simulink model "power_dstatcom_pwm"  (R2013a)
settings: Solver=FixedStepDiscrete  SolverMode=SingleTasking  StartTime=0.0  StopTime=0.5  FixedStep=Ts  RelTol=1e-3
InitFcn:
  |  Ts=5e-6;
undefined symbols (not defined in the file): D11, Delta, DiscIntNeverNeededParam
libraries: powerlib x39, powerlib_extras x25
(part 1 of 2)
Description:
  | Copyright 2008-2013 The MathWorks, Inc.
settings Model: ExtModeTrigMode=oneshot  ExtModeArmWhenConnect=off  ExtModeAutoUpdateStatusClock=off  Creator=MathWorks  LastModifiedBy=nau03113
settings DataIOCC: LimitDataPoints=off  SaveFinalState=on  SaveFormat=Structure  SignalLoggingSaveFormat=ModelDataLogs  SaveOutput=off  SaveTime=off  SignalLoggingName=sigsOut
settings OptimizationCC: BlockReduction=off  BooleanDataType=off  ExpressionDepthLimit=2147483647  InitFltsAndDblsToZero=on
settings DebuggingCC: SaveWithParameterizedLinksMsg=none  SignalResolutionControl=TryResolveAllWithWarning  SolverPrmCheckMsg=none  MultiTaskDSMMsg=warning  MultiTaskCondExecSysMsg=none  FcnCallInpInsideContextMsg=UseLocalSettings
settings HardwareCC: TargetUnknown=on
settings RTWCC: IncludeERTFirstTime=on
settings GRTTargetCC: TargetFcnLib=ansi_tfl_tmw.mat  CombineOutputUpdateFcns=off  GRTInterface=on

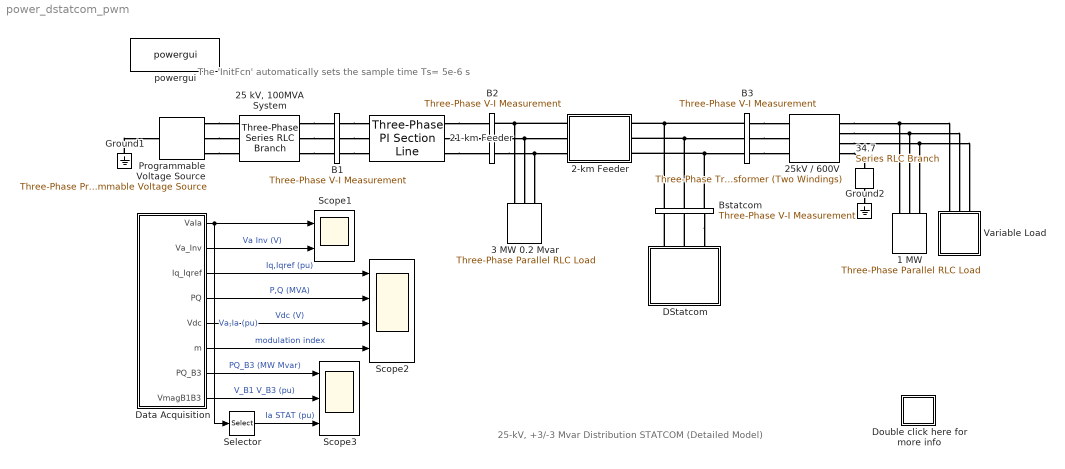
== system power_dstatcom_pwm ==
  note: The 'InitFcn' automatically sets
      |  the sample time Ts= 5e-6 s
  note: 25-kV, +3/-3 Mvar Distribution STATCOM (Detailed Model)
  1 MW : powerlib/Elements/Three-Phase Parallel RLC Load  LConnTagsString=A|B|C  Configuration=Y (floating)  NominalVoltage=600  NominalFrequency=60  ActivePower=1e6  InductivePower=0  CapacitivePower=0  Measurements=None  LoadType=constant Z
  2-km Feeder : Subsystem
      mask Display: plot(0,0,100,100,[20,20,80,80,90,80,80,20,20,10],[50,40,40,50,50,50,61,61,50,50])
  21-km Feeder : powerlib/Elements/Three-Phase PI Section Line  LConnTagsString=a|b|c  RConnTagsString=A|B|C  Frequency=60  Resistances=[0.1153 0.3963]  Inductances=[1.048e-3 2.730e-3]  Capacitances=[11.33e-9 5.338e-9]  Length=21
  "25 kV, 100MVA System" : powerlib/Elements/Three-Phase Series RLC Branch  LConnTagsString=A|B|C  RConnTagsString=A|B|C  BranchType=RL  Resistance=25e3^2/100e6/10  Inductance=25e3^2/100e6/(2*pi*60)  Capacitance=1.0  Measurements=None
  25kV / 600V : powerlib/Elements/Three-Phase Transformer (Two Windings)  Winding1Connection=Delta (D11)  UNITS=pu  NominalPower=[6e6 60]  Winding1=[25e3 , 0.05/30/2 , 0.05]  Winding2Connection=Yn  Winding2=[600 , 0.05/30/2 , 0]  SetSaturation=off  Rm=500  Lm=500  Saturation="[ 0,0  ;  0.005,1.2  ;  1.0,1.4 ]"  Hysteresis=off  DataFile='basic_model'  SetInitialFlux=off  InitialFluxes=[ 0.8 , -0.8 , 0.7 ]  Measurements=None  MoreParameters=off  BreakLoop=off  DataType=off  TransfoNumber=1
  3 MW 0.2 Mvar : powerlib/Elements/Three-Phase Parallel RLC Load  LConnTagsString=A|B|C  Configuration=Y (grounded)  NominalVoltage=25e3  NominalFrequency=60  ActivePower=3e6  InductivePower=0  CapacitivePower=0.2e6  Measurements=None  LoadType=constant Z
  34.7 : powerlib/Elements/Series RLC Branch  LConnTagsString=__new0  RConnTagsString=__new0  BranchType=R  Resistance=34.7  Inductance=1.0  SetiL0=off  InitialCurrent=0  Capacitance=1.0  Setx0=off  InitialVoltage=0  Measurements=None
  B1 : powerlib/Measurements/Three-Phase V-I Measurement  VoltageMeasurement=phase-to-ground  SetLabelV=on  LabelV=Vabc_B1  Vpu=on  VpuLL=off  CurrentMeasurement=no  SetLabelI=off  LabelI=A1  Ipu=off  Pbase=100e6  Vbase=25e3  OutputType=Magnitude  PhasorSimulation=off  PSBequivalent=0
  B2 : powerlib/Measurements/Three-Phase V-I Measurement  VoltageMeasurement=phase-to-ground  SetLabelV=on  LabelV=Vabc_B2  Vpu=on  VpuLL=off  CurrentMeasurement=no  SetLabelI=off  LabelI=Iabc_B2  Ipu=off  Pbase=3e6  Vbase=25e3  OutputType=Magnitude  PhasorSimulation=off  PSBequivalent=0
  B3 : powerlib/Measurements/Three-Phase V-I Measurement  VoltageMeasurement=phase-to-ground  SetLabelV=on  LabelV=Vabc_B3  Vpu=on  VpuLL=off  CurrentMeasurement=yes  SetLabelI=on  LabelI=Iabc_B3  Ipu=on  Pbase=1e6  Vbase=25e3  OutputType=Magnitude  PhasorSimulation=off  PSBequivalent=0
  Bstatcom : powerlib/Measurements/Three-Phase V-I Measurement  VoltageMeasurement=phase-to-ground  SetLabelV=on  LabelV=Vabc_Bstatcom  Vpu=on  VpuLL=off  CurrentMeasurement=yes  SetLabelI=on  LabelI=Iabc_Bstatcom  Ipu=on  Pbase=3e6  Vbase=25e3  OutputType=Magnitude  PhasorSimulation=off  PSBequivalent=0
  DStatcom : Subsystem
      mask Display: disp('D-STATCOM\n+/- 3Mvar')
  Data Acquisition : Subsystem
  Double click here for more info : Subsystem
      settings: OpenFcn=showdemo(bdroot(gcb))
      mask Display: disp('?')
  Ground1 : powerlib/Elements/Ground  LConnTagsString=a
  Ground2 : powerlib/Elements/Ground  LConnTagsString=a
  Programmable Voltage Source : powerlib/Electrical Sources/Three-Phase Programmable Voltage Source  PositiveSequence=[1.077*25e3 19 60]  VariationEntity=None  VariationType=Table of time-amplitude pairs  VariationTypeAlt=Step  VariationStep=0.5  VariationRate=10  VariationMagnitude=0.3  VariationFrequency=2  VariationTiming=[1 2]  VariationPhaseA=off  Amplitudes=[1 1.06 0.94 1.0]  TimeValues="[0 0.2  0.3   0.4 ]"  HarmonicGeneration=off  HarmonicA=[3 0.2 -25 0]  HarmonicB=[2 0.15 35 2]  Timing="[0.05  3]"  BusType=swing  Pref=0  Qref=0  Qmin=-inf  Qmax=inf
  Scope1 : Scope  NumInputPorts=2
      settings: TimeRange=0.5  YMin=-1.5~-4000  YMax=1.5~4000  SaveName=Sig1  SampleInput=on  SampleTime=Ts
  Scope2 : Scope  NumInputPorts=4
      settings: TimeRange=0.5  YMin=-1.5~-4~2200~0.4  YMax=1.5~4~2600~1.2  SaveName=Sig2  SampleInput=on  SampleTime=Ts*32
  Scope3 : Scope  NumInputPorts=3
      settings: TimeRange=0.5  YMin=0~0.9500000000000001~-1  YMax=6~1.15~1  SaveName=Sig  SampleInput=on  SampleTime=Ts
  Selector : Selector  InputPortWidth=2  IndexOptions=Index vector (dialog)  Indices=2  OutputSizes=1
  Variable Load : Subsystem  mask(Variable Load (Constant Current)){Par_Nom=[3000 0.9], Par_Mod=[2000  5], Par_Time=[0.15 1], Vbase=600, Ts=Ts}
      mask prompts: Par_Nom "Nominal load: [ Current (Arms)    Power factor (0 a 1) ]"; Par_Mod "Modulation: [ Amplitude (Arms)   Frequency (Hz) ]"; Par_Time "Modulation timing : [ Ton  Toff ]"; Vbase "Nominal voltage (Volts rms ph-ph)"; Ts "Sample time:"
      mask init:
      | NomAmp=Par_Nom(1)*sqrt(2);
      | NomPha=-acos(Par_Nom(2));
      | ModFreq=Par_Mod(2);
      | ModAmp=Par_Mod(1)*sqrt(2);
      | Ton=Par_Time(1);
      | Toff=Par_Time(2);
  powergui : powerlib/powergui  Priority=2  SimulationMode=Discrete  SolverType=Tustin  SampleTime=Ts  frequency=60  SPID=off  DisableSnubberDevices=off  DisableRonSwitches=off  DisableVfSwitches=off  SwTol=0  Interpol=off  DisplayEquations=off  frequencyindice=60  Pbase=100e6  ErrMax=1e-4  Iterations=50  UnitsV=kV  UnitsW=MW  FunctionMessages=off  echomessages=off  HookPort=off  EnableUseOfTLC=off  x0status=blocks  RestoreLinks=warning  ResistiveCurrentMeasurement=off  Frange=[0:2:500]  Ylog=off  Xlog=on  ShowGrid=off  save=off  variable=ZData  structure=Sig1  ZoomFFT=on  StartTime=0.26  cycles=2  DisplayStyle=1  fundamental=60  FreqAxis=off  MaxFrequency=5000  frequencyindicesteady=1  RmsSteady=1  display=off  Ts=0  methode=off
  wires:
  Data Acquisition/1(VaIa) -> Scope1/1, Selector/1  "Va,Ia (pu)"
  Data Acquisition/2(Va_Inv) -> Scope1/2  "Va Inv (V)"
  Data Acquisition/5(Vdc) -> Scope2/3  "Vdc (V)"
  Data Acquisition/4(PQ) -> Scope2/2  "P,Q (MVA)"
  Data Acquisition/3(Iq_Iqref) -> Scope2/1  "Iq,Iqref (pu)"
  Data Acquisition/6(m) -> Scope2/4  "modulation index"
  Selector/1 -> Scope3/3  "Ia STAT (pu)"
  Data Acquisition/7(PQ_B3) -> Scope3/1  "PQ_B3 (MW Mvar)"
  Data Acquisition/8(VmagB1B3) -> Scope3/2  "V_B1 V_B3 (pu)"
  connections:
  Bstatcom/LConn2 -- 2-km Feeder/RConn2 -- B3/LConn2
  B3/LConn1 -- Bstatcom/LConn1 -- 2-km Feeder/RConn1
  Bstatcom/LConn3 -- 2-km Feeder/RConn3 -- B3/LConn3
  34.7/RConn1 -- Ground2/LConn1
  25kV / 600V/RConn4 -- 34.7/LConn1
  25kV / 600V/RConn1 -- 1 MW/LConn1 -- Variable Load/LConn1
  25kV / 600V/RConn2 -- 1 MW/LConn2 -- Variable Load/LConn2
  25kV / 600V/RConn3 -- 1 MW/LConn3 -- Variable Load/LConn3
  Programmable Voltage Source/RConn1 -- "25 kV, 100MVA System"/LConn1
  Programmable Voltage Source/RConn2 -- "25 kV, 100MVA System"/LConn2
  Programmable Voltage Source/RConn3 -- "25 kV, 100MVA System"/LConn3
  Ground1/LConn1 -- Programmable Voltage Source/LConn1
  21-km Feeder/RConn1 -- B2/LConn1
  21-km Feeder/RConn2 -- B2/LConn2
  21-km Feeder/RConn3 -- B2/LConn3
  "25 kV, 100MVA System"/RConn1 -- B1/LConn1
  "25 kV, 100MVA System"/RConn2 -- B1/LConn2
  "25 kV, 100MVA System"/RConn3 -- B1/LConn3
  B1/RConn1 -- 21-km Feeder/LConn1
  B1/RConn2 -- 21-km Feeder/LConn2
  B1/RConn3 -- 21-km Feeder/LConn3
  2-km Feeder/LConn1 -- B2/RConn1 -- 3 MW 0.2 Mvar/LConn1
  B2/RConn2 -- 2-km Feeder/LConn2 -- 3 MW 0.2 Mvar/LConn2
  B2/RConn3 -- 2-km Feeder/LConn3 -- 3 MW 0.2 Mvar/LConn3
  Bstatcom/RConn3 -- DStatcom/RConn3
  DStatcom/RConn1 -- Bstatcom/RConn1
  DStatcom/RConn2 -- Bstatcom/RConn2
  B3/RConn1 -- 25kV / 600V/LConn1
  B3/RConn2 -- 25kV / 600V/LConn2
  B3/RConn3 -- 25kV / 600V/LConn3

== system power_dstatcom_pwm/2-km Feeder ==
  Three-Phase Mutual Inductance Z1-Z0 : powerlib/Elements/Three-Phase Mutual Inductance Z1-Z0  LConnTagsString=a|b|c  RConnTagsString=A|B|C  PositiveSequence="[0.1153  1.048e-3]*2"  ZeroSequence="[0.3963  2.730e-3]*2"
  A : PMIOPort  Port=1  Side=Left
  B : PMIOPort  Port=2  Side=Left
  "C " : PMIOPort  Port=3  Side=Left
  a : PMIOPort  Port=4  Side=Right
  b : PMIOPort  Port=5  Side=Right
  c : PMIOPort  Port=6  Side=Right
  connections:
  Three-Phase Mutual Inductance Z1-Z0/RConn3 -- c/RConn1
  Three-Phase Mutual Inductance Z1-Z0/RConn2 -- b/RConn1
  Three-Phase Mutual Inductance Z1-Z0/RConn1 -- a/RConn1
  "C "/RConn1 -- Three-Phase Mutual Inductance Z1-Z0/LConn3
  B/RConn1 -- Three-Phase Mutual Inductance Z1-Z0/LConn2
  A/RConn1 -- Three-Phase Mutual Inductance Z1-Z0/LConn1

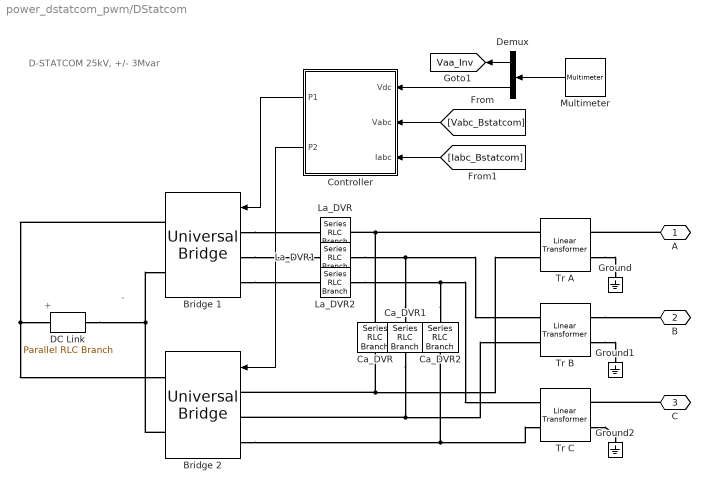
== system power_dstatcom_pwm/DStatcom ==
  note: +
  note: -
  note: D-STATCOM
      | 25kV, +/- 3Mvar
  "Bridge 1 " : powerlib/Power Electronics/Universal Bridge  Arms=3  SnubberResistance=1e5  SnubberCapacitance=inf  Device=IGBT / Diodes  Ron=1e-3  Lon=0  ForwardVoltages="[  2  0.8  ]"  ForwardVoltage=.8  GTOparameters=[ 10e-6 , 20e-6 ]  IGBTparameters=[ 0 0]  Measurements=Device voltages  Measurements_2=None  converterType=Rectifier
  Bridge 2 : powerlib/Power Electronics/Universal Bridge  Arms=3  SnubberResistance=1e5  SnubberCapacitance=inf  Device=IGBT / Diodes  Ron=1e-3  Lon=0  ForwardVoltages="[  2  0.8  ]"  ForwardVoltage=.8  GTOparameters=[ 10e-6 , 20e-6 ]  IGBTparameters=[ 0 0]  Measurements=Device voltages  Measurements_2=None  converterType=Rectifier
  Ca_DVR : powerlib/Elements/Series RLC Branch  LConnTagsString=__new0  RConnTagsString=__new0  BranchType=RC  Resistance=100e-6*(2*pi*60)/40  Inductance=1.0  SetiL0=off  InitialCurrent=0  Capacitance=100e-6  Setx0=off  InitialVoltage=0  Measurements=None
  Ca_DVR1 : powerlib/Elements/Series RLC Branch  LConnTagsString=__new0  RConnTagsString=__new0  BranchType=RC  Resistance=100e-6*(2*pi*60)/40  Inductance=1.0  SetiL0=off  InitialCurrent=0  Capacitance=100e-6  Setx0=off  InitialVoltage=0  Measurements=None
  Ca_DVR2 : powerlib/Elements/Series RLC Branch  LConnTagsString=__new0  RConnTagsString=__new0  BranchType=RC  Resistance=100e-6*(2*pi*60)/40  Inductance=1.0  SetiL0=off  InitialCurrent=0  Capacitance=100e-6  Setx0=off  InitialVoltage=0  Measurements=None
  Controller : Subsystem  mask(D-STATCOM Controller){ModeOper=Q regulation, Vac_Ref=1.0, Qref=0, Vdc_Ref=2400, Par_VacReg=[0.55 2500], Par_VdcReg=[0.001 0.15], Par_IReg=[0.8 200 0], Ts=Ts}
      mask prompts: ModeOper "Mode of operation:"; Vac_Ref "AC voltage setpoint Vref (pu):"; Qref "Manual mode: Qref (Reactive power in pu):"; Vdc_Ref "DC Voltage setpoint (Volts)"; Par_VacReg "Vac Regulator Gains: [ Kp  Ki ]"; Par_VdcReg "Vdc Regulator Gains: [ Kp  Ki ]"; Par_IReg "Current Regulators Gain: [ Kp Ki Kd ]"; Ts "Sample time (s)"
      mask init:
      | Kp_I=Par_IReg(1);
      | Ki_I=Par_IReg(2);
      | Kd_I=Par_IReg(3);
      | Kp_Vdc=Par_VdcReg(1);
      | Ki_Vdc=Par_VdcReg(2);
      | Kp_Vac=Par_VacReg(1);
      | Ki_Vac=Par_VacReg(2);
      mask TypeOptions ModeOper: Voltage regulation | Q regulation
  DC Link : powerlib/Elements/Parallel RLC Branch  LConnTagsString=a  RConnTagsString=__new0  BranchType=C  Resistance=1.0  Inductance=1.0  SetiL0=off  InitialCurrent=0  Capacitance=10000e-6  Setx0=off  InitialVoltage=0  Measurements=Branch voltage
  Demux : Demux  Outputs=[2 1 ]
  Ground : powerlib/Elements/Ground  LConnTagsString=a
  Ground1 : powerlib/Elements/Ground  LConnTagsString=a
  Ground2 : powerlib/Elements/Ground  LConnTagsString=a
  La_DVR : powerlib/Elements/Series RLC Branch  LConnTagsString=__new0  RConnTagsString=__new0  BranchType=L  Resistance=1.0  Inductance=800e-6  SetiL0=off  InitialCurrent=0  Capacitance=1.0  Setx0=off  InitialVoltage=0  Measurements=None
  La_DVR1 : powerlib/Elements/Series RLC Branch  LConnTagsString=__new0  RConnTagsString=__new0  BranchType=L  Resistance=1.0  Inductance=800e-6  SetiL0=off  InitialCurrent=0  Capacitance=1.0  Setx0=off  InitialVoltage=0  Measurements=None
  La_DVR2 : powerlib/Elements/Series RLC Branch  LConnTagsString=__new0  RConnTagsString=__new0  BranchType=L  Resistance=1.0  Inductance=800e-6  SetiL0=off  InitialCurrent=0  Capacitance=1.0  Setx0=off  InitialVoltage=0  Measurements=None
  Multimeter : powerlib/Measurements/Multimeter  Tag=PoWeRsYsTeMmEaSuReMeNt  PhasorSimulation=off  OutputType=Magnitude  sel=[3 9 1]  L=13  Gain=[1 1 1]  yselected={'Usw2: DStatcom/Bridge 1 ','Usw2: DStatcom/Bridge 2','Ub: DStatcom/DC Link'};  PSBOutputType=1  PSBequivalent=0  AxesSetting=[0,0.1,-100,100]  Display=0  SavedBlockNames=-11
      settings: AttributesFormatString=\n
  Tr A : powerlib/Elements/Linear Transformer  LConnTagsString=a|b  RConnTagsString=A|B  UNITS=pu  NominalPower=[3e6/3 60]  winding1=[1250 0.03/30 0.03]  winding2=[25e3/sqrt(3) 0.03/30 0.03]  ThreeWindings=off  winding3=[60e3 0.005 0.02]  RmLm=[200 200]  Measurements=None  DataType=off
  Tr B : powerlib/Elements/Linear Transformer  LConnTagsString=a|b  RConnTagsString=A|B  UNITS=pu  NominalPower=[3e6/3 60]  winding1=[1250 0.03/30 0.03]  winding2=[25e3/sqrt(3) 0.03/30 0.03]  ThreeWindings=off  winding3=[60e3 0.005 0.02]  RmLm=[200 200]  Measurements=None  DataType=off
  Tr C : powerlib/Elements/Linear Transformer  LConnTagsString=a|b  RConnTagsString=A|B  UNITS=pu  NominalPower=[3e6/3 60]  winding1=[1250 0.03/30 0.03]  winding2=[25e3/sqrt(3) 0.03/30 0.03]  ThreeWindings=off  winding3=[60e3 0.005 0.02]  RmLm=[200 200]  Measurements=None  DataType=off
  A : PMIOPort  Port=1  Side=Right
  B : PMIOPort  Port=2  Side=Right
  C : PMIOPort  Port=3  Side=Right
  tag scope: Vaa_Inv=global
  wires:
  Controller/1(P1) -> "Bridge 1 "/1
  Controller/2(P2) -> Bridge 2/1
  Multimeter/1 -> Demux/1
  Demux/2 -> Controller/1(Vdc)
  Demux/1 -> [Vaa_Inv]
  [Vabc_Bstatcom] -> Controller/2(Vabc)
  [Iabc_Bstatcom] -> Controller/3(Iabc)
  connections:
  "Bridge 1 "/LConn1 -- La_DVR/LConn1
  "Bridge 1 "/LConn2 -- La_DVR1/LConn1
  "Bridge 1 "/LConn3 -- La_DVR2/LConn1
  Bridge 2/LConn2 -- Tr B/LConn2 -- Ca_DVR1/LConn1
  Bridge 2/LConn3 -- Tr C/LConn2 -- Ca_DVR2/LConn1
  Ca_DVR1/RConn1 -- La_DVR1/RConn1 -- Tr B/LConn1
  Ca_DVR2/RConn1 -- La_DVR2/RConn1 -- Tr C/LConn1
  Tr A/LConn1 -- La_DVR/RConn1 -- Ca_DVR/RConn1
  Tr C/RConn2 -- Ground2/LConn1
  Tr B/RConn2 -- Ground1/LConn1
  Tr A/RConn2 -- Ground/LConn1
  A/RConn1 -- Tr A/RConn1
  Tr B/RConn1 -- B/RConn1
  C/RConn1 -- Tr C/RConn1
  "Bridge 1 "/RConn1 -- Bridge 2/RConn1 -- DC Link/LConn1
  Bridge 2/RConn2 -- "Bridge 1 "/RConn2 -- DC Link/RConn1
  Bridge 2/LConn1 -- Tr A/LConn2 -- Ca_DVR/LConn1

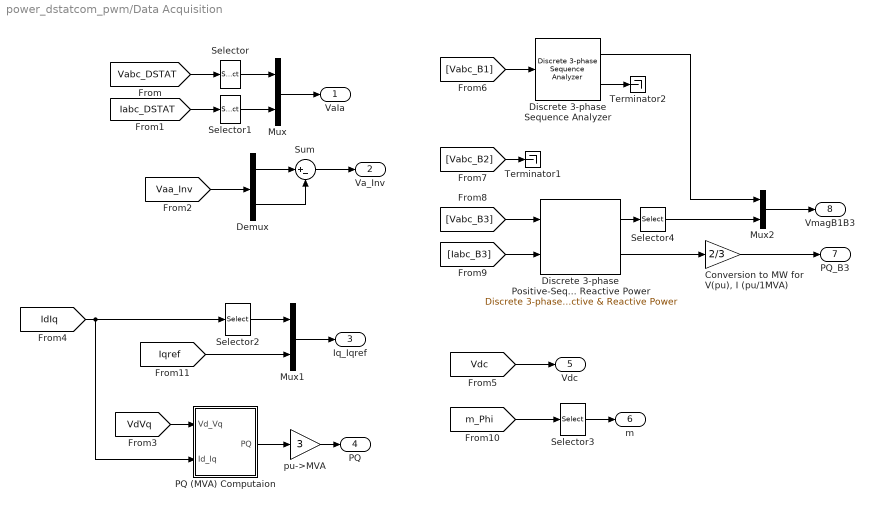
== system power_dstatcom_pwm/Data Acquisition ==
  "Conversion to MW for V(pu), I (pu/1MVA)" : Gain  Gain=2/3  SaturateOnIntegerOverflow=on  OutDataTypeStr=Inherit: Same as input  ParamDataTypeStr=Inherit: Same as input
  Demux : Demux  Outputs=2
  Discrete 3-phase Sequence Analyzer : powerlib_extras/Discrete Measurements/Discrete 3-phase Sequence Analyzer  Freq=60  n=1  seq=Positive  Par_Init=[1 0]  Ts=Ts
  Discrete 3-phase Positive-Sequence Active & Reactive Power : powerlib_extras/Discrete Measurements/Discrete 3-phase  Positive-Sequence  Active & Reactive Power  Freq=60  Par_Vinit=[1 0]  Par_Iinit=[0 0]  Ts=Ts
  Mux : Mux  Inputs=2
  Mux1 : Mux  Inputs=2
  Mux2 : Mux  Inputs=2
  PQ (MVA) Computaion : Subsystem
  Selector : Selector  InputPortWidth=3  IndexOptions=Index vector (dialog)  Indices=1  OutputSizes=1
  Selector1 : Selector  InputPortWidth=3  IndexOptions=Index vector (dialog)  Indices=1  OutputSizes=1
  Selector2 : Selector  InputPortWidth=2  IndexOptions=Index vector (dialog)  Indices=2  OutputSizes=1
  Selector3 : Selector  InputPortWidth=2  IndexOptions=Index vector (dialog)  Indices=1  OutputSizes=1
  Selector4 : Selector  InputPortWidth=2  IndexOptions=Index vector (dialog)  Indices=1  OutputSizes=1
  Sum : Sum  Inputs=|+-  SaturateOnIntegerOverflow=on
  Terminator1 : Terminator
  Terminator2 : Terminator
  pu->MVA : Gain  Gain=3  SaturateOnIntegerOverflow=on  OutDataTypeStr=Inherit: Same as input  ParamDataTypeStr=Inherit: Same as input
  VaIa : Outport
  Va_Inv : Outport  Port=2
  Iq_Iqref : Outport  Port=3
  PQ : Outport  Port=4
  Vdc : Outport  Port=5
  m : Outport  Port=6
  PQ_B3 : Outport  Port=7
  VmagB1B3 : Outport  Port=8
  wires:
  [Vdc] -> Vdc/1
  [IdIq] -> Selector2/1, PQ (MVA) Computaion/2(Id_Iq)
  Selector/1 -> Mux/1
  Selector1/1 -> Mux/2
  Mux/1 -> VaIa/1
  [m_Phi] -> Selector3/1
  [Vabc_DSTAT] -> Selector/1
  [Iabc_DSTAT] -> Selector1/1
  Mux1/1 -> Iq_Iqref/1
  Selector2/1 -> Mux1/1
  [Iqref] -> Mux1/2
  PQ (MVA) Computaion/1(PQ) -> pu->MVA/1
  pu->MVA/1 -> PQ/1
  [VdVq] -> PQ (MVA) Computaion/1(Vd_Vq)
  Selector3/1 -> m/1
  [Vaa_Inv] -> Demux/1
  Demux/1 -> Sum/1
  Demux/2 -> Sum/2
  Sum/1 -> Va_Inv/1
  [Vabc_B2] -> Terminator1/1
  [Vabc_B3] -> Discrete 3-phase Positive-Sequence Active & Reactive Power/1
  [Iabc_B3] -> Discrete 3-phase Positive-Sequence Active & Reactive Power/2
  Discrete 3-phase Positive-Sequence Active & Reactive Power/2 -> "Conversion to MW for V(pu), I (pu/1MVA)"/1
  [Vabc_B1] -> Discrete 3-phase Sequence Analyzer/1
  Discrete 3-phase Sequence Analyzer/1 -> Mux2/1
  Mux2/1 -> VmagB1B3/1
  "Conversion to MW for V(pu), I (pu/1MVA)"/1 -> PQ_B3/1
  Discrete 3-phase Positive-Sequence Active & Reactive Power/1 -> Selector4/1
  Selector4/1 -> Mux2/2
  Discrete 3-phase Sequence Analyzer/2 -> Terminator2/1

== system power_dstatcom_pwm/Double click here for more info ==

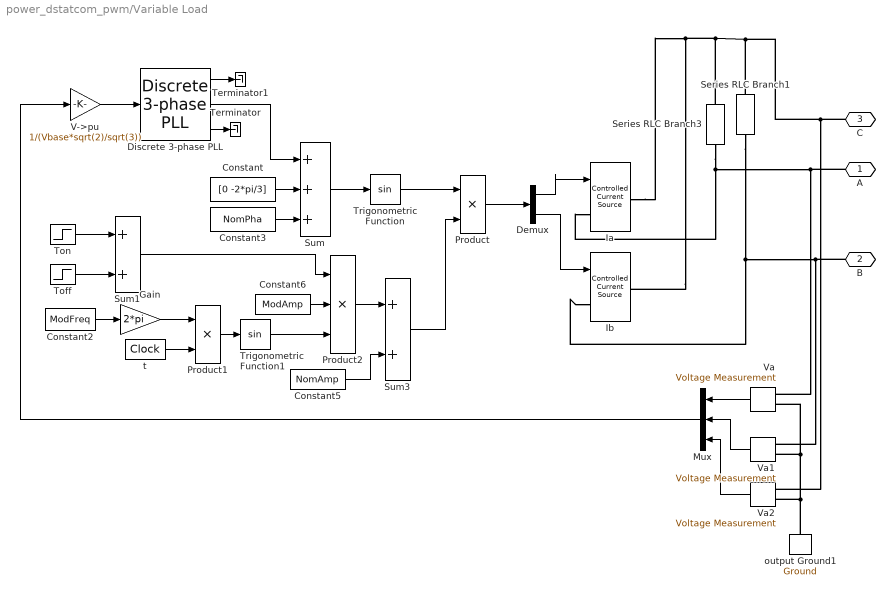
== system power_dstatcom_pwm/Variable Load ==
  Constant : Constant  Value=[0 -2*pi/3]
  Constant2 : Constant  Value=ModFreq
  Constant3 : Constant  Value=NomPha
  Constant5 : Constant  Value=NomAmp
  Constant6 : Constant  Value=ModAmp
  Demux : Demux  Outputs=2
  Discrete 3-phase PLL : powerlib_extras/Discrete  Control Blocks/Discrete 3-phase PLL  Fmin=45  Par_Init=[0 60]  ParK=[60 1400]  Ts=Ts  AGC=off
  Gain : Gain  Gain=2*pi  SaturateOnIntegerOverflow=on  OutDataTypeStr=Inherit: Same as input  ParamDataTypeStr=Inherit: Same as input
  Ia : powerlib/Electrical Sources/Controlled Current Source  Description=source block  Initialize=on  Source_Type=AC  Amplitude=0  Phase=0  Frequency=0  Measurements=None
      settings: AttributesFormatString=\n
  Ib : powerlib/Electrical Sources/Controlled Current Source  Description=source block  Initialize=on  Source_Type=AC  Amplitude=0  Phase=0  Frequency=0  Measurements=None
      settings: AttributesFormatString=\n
  Mux : Mux  Inputs=3
  Product : Product  SaturateOnIntegerOverflow=on  InputSameDT=on  OutDataTypeStr=Inherit: Same as first input
  Product1 : Product  SaturateOnIntegerOverflow=on  InputSameDT=on  OutDataTypeStr=Inherit: Same as first input
  Product2 : Product  Inputs=3  SaturateOnIntegerOverflow=on  InputSameDT=on  OutDataTypeStr=Inherit: Same as first input
  Series RLC Branch1 : powerlib/Elements/Series RLC Branch  LConnTagsString=__new0  RConnTagsString=__new0  BranchType=R  Resistance=1e6  Inductance=1.0  SetiL0=off  InitialCurrent=0  Capacitance=1.0  Setx0=off  InitialVoltage=0  Measurements=None
  Series RLC Branch3 : powerlib/Elements/Series RLC Branch  LConnTagsString=__new0  RConnTagsString=__new0  BranchType=R  Resistance=1e6  Inductance=1.0  SetiL0=off  InitialCurrent=0  Capacitance=1.0  Setx0=off  InitialVoltage=0  Measurements=None
  Sum : Sum  Inputs=+++  SaturateOnIntegerOverflow=on  InputSameDT=on  OutDataTypeStr=Inherit: Same as first input
  Sum1 : Sum  SaturateOnIntegerOverflow=on  InputSameDT=on  OutDataTypeStr=Inherit: Same as first input
  Sum3 : Sum  SaturateOnIntegerOverflow=on  InputSameDT=on  OutDataTypeStr=Inherit: Same as first input
  Terminator : Terminator
  Terminator1 : Terminator
  Toff : Step  Time=Toff  After=-1  SampleTime=Ts
  Ton : Step  Time=Ton  SampleTime=Ts
  Trigonometric Function : Trigonometry
  Trigonometric Function1 : Trigonometry
  V->pu : Gain  Gain=1/(Vbase*sqrt(2)/sqrt(3))  SaturateOnIntegerOverflow=on  OutDataTypeStr=Inherit: Same as input  ParamDataTypeStr=Inherit: Same as input
  Va : powerlib/Measurements/Voltage Measurement  Tag=PoWeRsYsTeMmEaSuReMeNt  PhasorSimulation=off  OutputType=Magnitude  PSBequivalent=0
  Va1 : powerlib/Measurements/Voltage Measurement  Tag=PoWeRsYsTeMmEaSuReMeNt  PhasorSimulation=off  OutputType=Magnitude  PSBequivalent=0
  Va2 : powerlib/Measurements/Voltage Measurement  Tag=PoWeRsYsTeMmEaSuReMeNt  PhasorSimulation=off  OutputType=Magnitude  PSBequivalent=0
  output Ground1 : powerlib/Elements/Ground  LConnTagsString=a  RConnTagsString=__newr0
  t : DigitalClock  SampleTime=Ts
  A : PMIOPort  Port=1  Side=Left
  B : PMIOPort  Port=2  Side=Left
  C : PMIOPort  Port=3  Side=Left
  wires:
  Sum1/1 -> Product2/1
  Toff/1 -> Sum1/2
  Ton/1 -> Sum1/1
  Constant6/1 -> Product2/2
  Trigonometric Function1/1 -> Product2/3
  Constant5/1 -> Sum3/2
  Product2/1 -> Sum3/1
  Sum3/1 -> Product/2
  Product1/1 -> Trigonometric Function1/1
  t/1 -> Product1/2
  Gain/1 -> Product1/1
  Constant2/1 -> Gain/1
  Constant3/1 -> Sum/3
  Mux/1 -> V->pu/1
  Discrete 3-phase PLL/2 -> Sum/1
  V->pu/1 -> Discrete 3-phase PLL/1
  Discrete 3-phase PLL/3 -> Terminator/1
  Discrete 3-phase PLL/1 -> Terminator1/1
  Product/1 -> Demux/1
  Trigonometric Function/1 -> Product/1
  Sum/1 -> Trigonometric Function/1
  Constant/1 -> Sum/2
  Va2/1 -> Mux/3
  Va1/1 -> Mux/2
  Va/1 -> Mux/1
  Demux/2 -> Ib/1
  Demux/1 -> Ia/1
  connections:
  output Ground1/LConn1 -- Va2/LConn2 -- Va1/LConn2 -- Va/LConn2
  Ib/LConn1 -- Series RLC Branch1/LConn1 -- B/RConn1 -- Va1/LConn1
  Ia/LConn1 -- Series RLC Branch3/LConn1 -- A/RConn1 -- Va/LConn1
  Series RLC Branch1/RConn1 -- Series RLC Branch3/RConn1 -- Ia/RConn1 -- Ib/RConn1 -- C/RConn1 -- Va2/LConn1

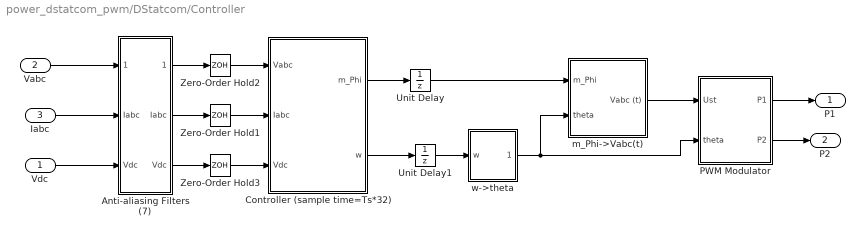
== system power_dstatcom_pwm/DStatcom/Controller ==
  Vdc : Inport  PortDimensions=1
  Vabc : Inport  Port=2  PortDimensions=3
  Iabc : Inport  Port=3  PortDimensions=3
  Anti-aliasing Filters (7) : Subsystem  mask(Anti-aliasing (2nd order lowpass)){Fc=2000, Ts=Ts}
      mask prompts: Fc "Cut-off frequency (Hz):"; Ts "Sample time:"
  Controller (sample time=Ts*32) : Subsystem
  "PWM Modulator " : Subsystem  mask(2- or 3- level, 3-phase PWM modulator){ModulatorType=2-level, ModulatorMode=Synchronized, nF=28, ModulatingSignals=External, Fc=28*60, m=0.75, Freq=60, Phase=0, Ts=Ts}
      mask prompts: ModulatorType "Type"; ModulatorMode "Mode of operation"; nF "Switching ratio: chopping frequency / output frequency"; ModulatingSignals "Modulating signal(s) for un-synchronized mode:"; Fc "Carrier frequency (Hz):"; m "Modulation Index:"; Freq "Output voltage frequency (Hz):"; Phase "Output voltage phase (degrees):"; Ts "Sample time:"
      mask init:
      | if ModulatorType==1
      |     nPulses=6;
      |     SelectorElements=[1:1:12];
      | else
      |     nPulses=12;
      |  SelectorElements=[1:1:24];
      | end
      mask TypeOptions ModulatorType: 2-level | 3-level
      mask TypeOptions ModulatorMode: Synchronized | Un-synchronized
      mask TypeOptions ModulatingSignals: External | Internal
  Unit Delay : UnitDelay  SampleTime=Ts*32
  Unit Delay1 : UnitDelay  SampleTime=Ts*32
  Zero-Order Hold1 : ZeroOrderHold  SampleTime=Ts*32
  Zero-Order Hold2 : ZeroOrderHold  SampleTime=Ts*32
  Zero-Order Hold3 : ZeroOrderHold  SampleTime=Ts*32
  m_Phi->Vabc(t) : Subsystem
  w->theta : Subsystem
  P1 : Outport
  P2 : Outport  Port=2
  wires:
  w->theta/1(theta) -> "PWM Modulator "/2(theta), m_Phi->Vabc(t)/2(theta)
  Unit Delay1/1 -> w->theta/1(w)
  Controller (sample time=Ts*32)/2(w) -> Unit Delay1/1
  m_Phi->Vabc(t)/1(Vabc (t)) -> "PWM Modulator "/1(Ust)
  Unit Delay/1 -> m_Phi->Vabc(t)/1(m_Phi)
  Controller (sample time=Ts*32)/1(m_Phi) -> Unit Delay/1
  Zero-Order Hold3/1 -> Controller (sample time=Ts*32)/3(Vdc)
  "PWM Modulator "/2(P2) -> P2/1
  "PWM Modulator "/1(P1) -> P1/1
  Zero-Order Hold1/1 -> Controller (sample time=Ts*32)/2(Iabc)
  Zero-Order Hold2/1 -> Controller (sample time=Ts*32)/1(Vabc)
  Vdc/1 -> Anti-aliasing Filters (7)/3("Vdc ")
  Iabc/1 -> Anti-aliasing Filters (7)/2("Iabc ")
  Vabc/1 -> Anti-aliasing Filters (7)/1(Vabc)
  Anti-aliasing Filters (7)/3(" Vdc") -> Zero-Order Hold3/1
  Anti-aliasing Filters (7)/2(Iabc) -> Zero-Order Hold1/1
  Anti-aliasing Filters (7)/1(" Vabc") -> Zero-Order Hold2/1

== system power_dstatcom_pwm/Data Acquisition/PQ (MVA) Computaion ==
  note: PQ Measurement:
  note: Q = Vq*Id-Vd*Iq
  note: P = Vd*Id + Vq*Iq
  Vd_Vq : Inport  PortDimensions=2
  Id_Iq : Inport  Port=2  PortDimensions=2
  Demux1 : Demux  Outputs=2
  Demux2 : Demux  Outputs=2
  Mux2 : Mux  Inputs=2
  Product{2..5} (4 alike) : Product  SaturateOnIntegerOverflow=on  InputSameDT=on  OutDataTypeStr=Inherit: Same as first input
  Sum : Sum  SaturateOnIntegerOverflow=on  InputSameDT=on  OutDataTypeStr=Inherit: Same as first input
  Sum1 : Sum  Inputs=+-  SaturateOnIntegerOverflow=on  InputSameDT=on  OutDataTypeStr=Inherit: Same as first input
  PQ : Outport
  wires:
  Demux2/2 -> Product5/2, Product3/2
  Demux1/1 -> Product5/1, Product2/1
  Demux2/1 -> Product4/2, Product2/2
  Demux1/2 -> Product4/1, Product3/1
  Id_Iq/1 -> Demux2/1
  Vd_Vq/1 -> Demux1/1
  Sum1/1 -> Mux2/2
  Sum/1 -> Mux2/1
  Product5/1 -> Sum1/2
  Product4/1 -> Sum1/1
  Product3/1 -> Sum/2
  Product2/1 -> Sum/1
  Mux2/1 -> PQ/1

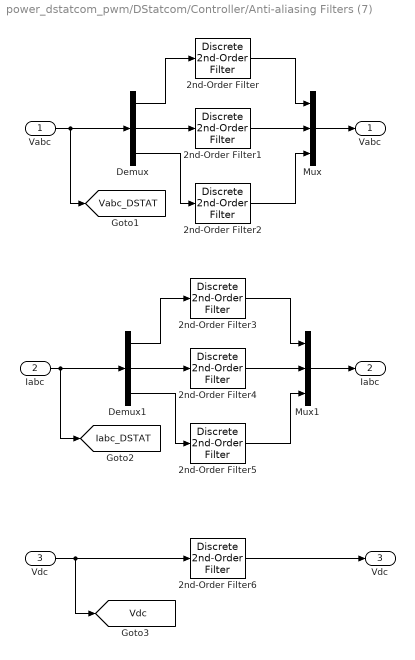
== system power_dstatcom_pwm/DStatcom/Controller/Anti-aliasing Filters (7) ==
  Vabc : Inport  PortDimensions=3
  "Iabc " : Inport  Port=2  PortDimensions=3
  "Vdc " : Inport  Port=3  PortDimensions=1
  2nd-Order Filter{,1..6} (7 alike) : powerlib_extras/Discrete  Control Blocks/Discrete  2nd-Order Filter  FilterType=Lowpass  Fo=Fc  Zeta=0.707  Ts=Ts  Initialize=off  Vac_Init=[0.8 -25 60]  Vdc_Init=-0.4  PlotResponse=off  param1=[1 5000 0.1]
  Demux : Demux  Outputs=3
  Demux1 : Demux  Outputs=3
  Mux : Mux  Inputs=3
  Mux1 : Mux  Inputs=3
  " Vabc" : Outport
  Iabc : Outport  Port=2
  " Vdc" : Outport  Port=3
  tag scope: Iabc_DSTAT=global, Vabc_DSTAT=global, Vdc=global
  wires:
  "Iabc "/1 -> Demux1/1, [Iabc_DSTAT]
  Demux1/2 -> 2nd-Order Filter4/1
  Demux1/3 -> 2nd-Order Filter5/1
  2nd-Order Filter5/1 -> Mux1/3
  2nd-Order Filter4/1 -> Mux1/2
  Mux1/1 -> Iabc/1
  2nd-Order Filter3/1 -> Mux1/1
  Demux1/1 -> 2nd-Order Filter3/1
  Demux/2 -> 2nd-Order Filter1/1
  Demux/3 -> 2nd-Order Filter2/1
  2nd-Order Filter2/1 -> Mux/3
  2nd-Order Filter1/1 -> Mux/2
  2nd-Order Filter6/1 -> " Vdc"/1
  "Vdc "/1 -> 2nd-Order Filter6/1, [Vdc]
  Mux/1 -> " Vabc"/1
  2nd-Order Filter/1 -> Mux/1
  Vabc/1 -> Demux/1, [Vabc_DSTAT]
  Demux/1 -> 2nd-Order Filter/1

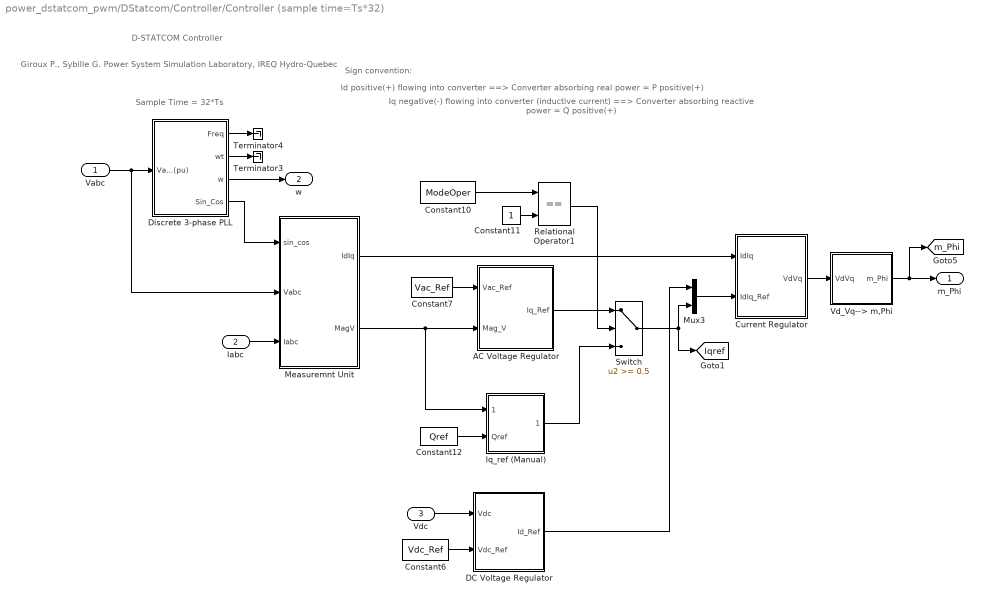
== system power_dstatcom_pwm/DStatcom/Controller/Controller (sample time=Ts*32) ==
  note: D-STATCOM Controller
  note: Giroux P., Sybille G.
      | Power System Simulation Laboratory, IREQ
      | Hydro-Quebec
  note: Iq negative(-) flowing into converter (inductive current) ==> Converter absorbing reactive power = Q positive(+)
  note: Sign convention:
  note: Id positive(+) flowing into converter ==> Converter absorbing real power = P positive(+)
  note: Sample Time = 32*Ts
  Vabc : Inport  PortDimensions=3
  Iabc : Inport  Port=2  PortDimensions=3
  Vdc : Inport  Port=3  PortDimensions=1
  AC Voltage Regulator : Subsystem  mask(DC Voltage regulator){Kp=Kp_Vac, Ki=Ki_Vac, Ts=32*Ts}
      mask prompts: Kp "Proportional gain (Kp):"; Ki "Integral gain(Ki)"; Ts "Sample time:"
  Constant10 : Constant  Value=ModeOper
  Constant11 : Constant
  Constant12 : Constant  Value=Qref
  Constant6 : Constant  Value=Vdc_Ref
  Constant7 : Constant  Value=Vac_Ref
  Current Regulator : Subsystem  mask(Current Regulators){Kp=Kp_I, Ki=Ki_I, Kd=Kd_I, TcD=0.2e-3, Par_Limits=[1 -1], Init=0, Ts=32*Ts}
      mask prompts: Kp "Proportional gain (Kp):"; Ki "Integral gain (Ki):"; Kd "Derivative gain (Kd):"; TcD "Time constant for derivative (s):"; Par_Limits "Output limits: [ Upper   Lower ]"; Init "Output initial value:"; Ts "Sample time:"
      mask help:
      | Sign convention:
      | Id positive(+) flowing into converter ==> Converter absorbing real power = P positive(+)
      | Iq negative(-) flowing into converter (inductive current) ==> Converter absorbing reactive power = Q positive(+)
  DC Voltage Regulator : Subsystem  mask(DC Voltage regulator){Kp=Kp_Vdc, Ki=Ki_Vdc, Ts=32*Ts}
      mask prompts: Kp "Proportional gain (Kp):"; Ki "Integral gain(Ki)"; Ts "Sample time:"
  Discrete 3-phase PLL : Subsystem  mask(Discrete 3-phase PLL){Par_Init=[3.7 60], ParK=[60 1400], Ts=32*Ts}
      mask prompts: Par_Init "Initial inputs:[ Phase(degrees)   Frequency(Hz) ]"; ParK "Regulator gains [ Kp  Ki ]"; Ts "Sample time:"
      mask help:
      | This Phase Locked Loop (PLL) system can be used  to synchronize on a set of variable frequency, three-phase sinusoidal signals.
      |
      | Input 1: Vector containing the normalized
      |              three-phase signals [Va Vb Vc]
      | Output 1:  Measured frequency (Hz) = w/(2pi)
      | Output 2:  Ramp w.t   varying between  0 and 2*pi,
      | synchronized on zero crossings of the fundamental (positive-sequence) of phase A.
      | Output 3: Vector [sin(wt) cos(wt)]
      mask init:
      | Kp=ParK(1);
      | Ki=ParK(2);
      | Phase_Init=Par_Init(1);
      | Finit=Par_Init(2);
  Iq_ref (Manual) : Subsystem
  Measuremnt Unit : Subsystem
  Mux3 : Mux  Inputs=2
  Relational Operator1 : RelationalOperator  Operator===  InputSameDT=on
  Switch : Switch  Threshold=0.5  SaturateOnIntegerOverflow=on  InputSameDT=on
  Terminator3 : Terminator
  Terminator4 : Terminator
  Vd_Vq--> m,Phi : Subsystem
  m_Phi : Outport
  w : Outport  Port=2
  tag scope: Iqref=global, m_Phi=global
  wires:
  Vd_Vq--> m,Phi/1(m_Phi) -> [m_Phi], m_Phi/1
  Current Regulator/1(VdVq) -> Vd_Vq--> m,Phi/1(VdVq)
  Relational Operator1/1 -> Switch/2
  Iq_ref (Manual)/1(Iqref*) -> Switch/3
  DC Voltage Regulator/1(Id_Ref) -> Mux3/1
  Switch/1 -> [Iqref], Mux3/2
  Mux3/1 -> Current Regulator/2(IdIq_Ref)
  AC Voltage Regulator/1(Iq_Ref) -> Switch/1
  Measuremnt Unit/1(IdIq) -> Current Regulator/1(IdIq)
  Constant7/1 -> AC Voltage Regulator/1(Vac_Ref)
  Measuremnt Unit/2(MagV) -> Iq_ref (Manual)/1(MagV), AC Voltage Regulator/2(Mag_V)
  Iabc/1 -> Measuremnt Unit/3(Iabc)
  Discrete 3-phase PLL/4(Sin_Cos) -> Measuremnt Unit/1(sin_cos)
  Discrete 3-phase PLL/3(w) -> w/1
  Discrete 3-phase PLL/1(Freq) -> Terminator4/1
  Discrete 3-phase PLL/2(wt) -> Terminator3/1
  Constant12/1 -> Iq_ref (Manual)/2(Qref)
  Constant10/1 -> Relational Operator1/1
  Constant11/1 -> Relational Operator1/2
  Vdc/1 -> DC Voltage Regulator/1(Vdc)
  Constant6/1 -> DC Voltage Regulator/2(Vdc_Ref)
  Vabc/1 -> Measuremnt Unit/2(Vabc), Discrete 3-phase PLL/1(Vabc (pu))

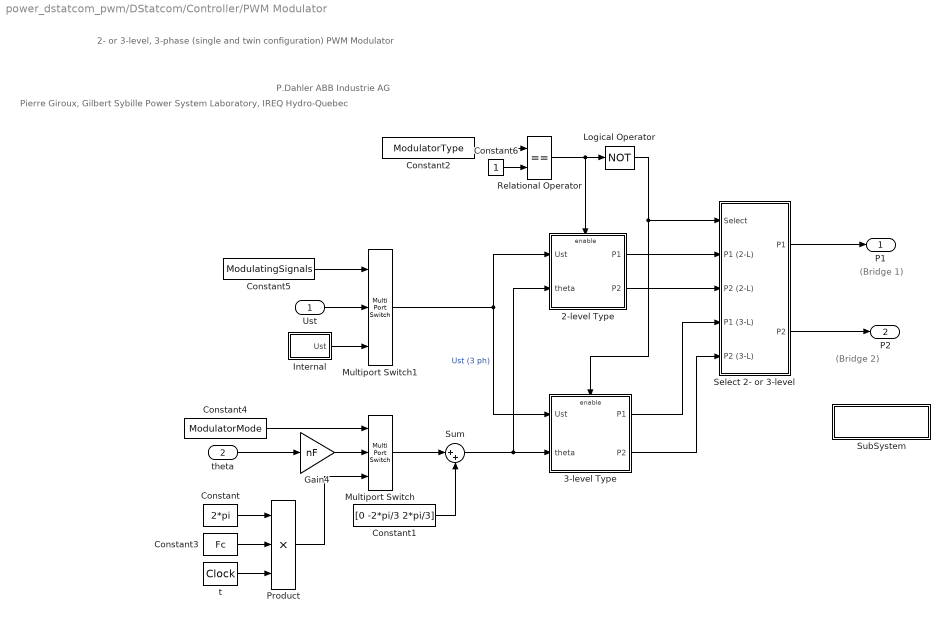
== system power_dstatcom_pwm/DStatcom/Controller/PWM Modulator  ==
  note: P.Dahler
      | ABB Industrie AG
  note: (Bridge 1)
  note: (Bridge 2)
  note: 2- or 3-level, 3-phase
      | (single and twin configuration)
      | PWM Modulator
  note: Pierre Giroux, Gilbert Sybille
      | Power System Laboratory, IREQ
      | Hydro-Quebec
  Ust : Inport  PortDimensions=3
  theta : Inport  Port=2  PortDimensions=1
  2-level Type : Subsystem  TreatAsAtomicUnit=on
  3-level Type : Subsystem  TreatAsAtomicUnit=on
  Constant : Constant  Value=2*pi
  Constant1 : Constant  Value=[0 -2*pi/3 2*pi/3]
  Constant2 : Constant  Value=ModulatorType
  Constant3 : Constant  Value=Fc
  Constant4 : Constant  Value=ModulatorMode
  Constant5 : Constant  Value=ModulatingSignals
  Constant6 : Constant
  Gain4 : Gain  Gain=nF  SaturateOnIntegerOverflow=on  OutDataTypeStr=Inherit: Same as input  ParamDataTypeStr=Inherit: Same as input
  Internal : Subsystem  mask(3-ph signal generator){m=m, Freq=Freq, Phase=Phase, Ts=Ts}
      mask prompts: m "Modulation Index:"; Freq "Output signal frequency (Hz):"; Phase "Output signal phase (degrees):"; Ts "Sample time:"
  Logical Operator : Logic  Operator=NOT
  Multiport Switch : MultiPortSwitch  Inputs=2  SaturateOnIntegerOverflow=on  InputSameDT=on
  Multiport Switch1 : MultiPortSwitch  Inputs=2  SaturateOnIntegerOverflow=on  InputSameDT=on
  Product : Product  Inputs=3  SaturateOnIntegerOverflow=on  InputSameDT=on  OutDataTypeStr=Inherit: Same as first input
  Relational Operator : RelationalOperator  Operator===  InputSameDT=on
  Select 2- or 3-level : Subsystem
  SubSystem : Subsystem
      mask Display: disp('Pulse pattern\ndescription')
  Sum : Sum  Inputs=|++  SaturateOnIntegerOverflow=on  InputSameDT=on  OutDataTypeStr=Inherit: Same as first input
  t : DigitalClock  SampleTime=Ts
  P1 : Outport
  P2 : Outport  Port=2
  wires:
  2-level Type/2(P2) -> Select 2- or 3-level/3(P2 (2-L))
  2-level Type/1(P1) -> Select 2- or 3-level/2(P1 (2-L))
  Select 2- or 3-level/1(P1) -> P1/1
  Select 2- or 3-level/2(P2) -> P2/1
  3-level Type/2(P2) -> Select 2- or 3-level/5(P2 (3-L))
  3-level Type/1(P1) -> Select 2- or 3-level/4(P1 (3-L))
  Logical Operator/1 -> Select 2- or 3-level/1(Select), 3-level Type/Enable
  Constant2/1 -> Relational Operator/1
  Relational Operator/1 -> Logical Operator/1, 2-level Type/Enable
  Constant6/1 -> Relational Operator/2
  Sum/1 -> 3-level Type/2(theta), 2-level Type/2(theta)
  Multiport Switch1/1 -> 3-level Type/1(Ust), 2-level Type/1(Ust)  "Ust (3 ph)"
  Constant1/1 -> Sum/2
  Multiport Switch/1 -> Sum/1
  Constant/1 -> Product/1
  Constant3/1 -> Product/2
  t/1 -> Product/3
  theta/1 -> Gain4/1
  Constant4/1 -> Multiport Switch/1
  Gain4/1 -> Multiport Switch/2
  Product/1 -> Multiport Switch/3
  Internal/1(Ust) -> Multiport Switch1/3
  Constant5/1 -> Multiport Switch1/1
  Ust/1 -> Multiport Switch1/2

== system power_dstatcom_pwm/DStatcom/Controller/m_Phi->Vabc(t) ==
  m_Phi : Inport
  theta : Inport  Port=2
  Constant1 : Constant  Value=[0 -2*pi/3 2*pi/3]
  Demux : Demux  Outputs=2
  Product2 : Product  SaturateOnIntegerOverflow=on  InputSameDT=on  OutDataTypeStr=Inherit: Same as first input
  Sum4 : Sum  Inputs=+++  SaturateOnIntegerOverflow=on  InputSameDT=on  OutDataTypeStr=Inherit: Same as first input
  Trigonometric Function1 : Trigonometry
  deg. ->rad : Gain  Gain=pi/180  SaturateOnIntegerOverflow=on  OutDataTypeStr=Inherit: Same as input  ParamDataTypeStr=Inherit: Same as input
  Vabc (t) : Outport
  wires:
  Demux/2 -> deg. ->rad/1
  theta/1 -> Sum4/3
  deg. ->rad/1 -> Sum4/1
  m_Phi/1 -> Demux/1
  Product2/1 -> Vabc (t)/1
  Demux/1 -> Product2/1
  Constant1/1 -> Sum4/2
  Sum4/1 -> Trigonometric Function1/1
  Trigonometric Function1/1 -> Product2/2

== system power_dstatcom_pwm/DStatcom/Controller/w->theta ==
  w : Inport
  Constant4 : Constant  Value=2*pi
  Discrete-Time Integrator : DiscreteIntegrator  SampleTime=Ts  ICPrevOutput=DiscIntNeverNeededParam  ICPrevScaledInput=DiscIntNeverNeededParam
  Math Function : Math  Operator=mod  SaturateOnIntegerOverflow=on
  theta : Outport
  wires:
  Math Function/1 -> theta/1
  w/1 -> Discrete-Time Integrator/1
  Constant4/1 -> Math Function/2
  Discrete-Time Integrator/1 -> Math Function/1

== system power_dstatcom_pwm/DStatcom/Controller/Controller (sample time=Ts*32)/AC Voltage Regulator ==
  Vac_Ref : Inport
  Mag_V : Inport  Port=2
  Discrete PI Controller : powerlib_extras/Discrete  Control Blocks/Discrete PI Controller  Kp=Kp  Ki=Ki  Par_Limits=[1 -1]  Init=0  Ts=Ts
  Sum : Sum  Inputs=|+-  SaturateOnIntegerOverflow=on  InputSameDT=on  OutDataTypeStr=Inherit: Same as first input
  Iq_Ref : Outport  InitialOutput=0
  wires:
  Sum/1 -> Discrete PI Controller/1
  Vac_Ref/1 -> Sum/1
  Mag_V/1 -> Sum/2
  Discrete PI Controller/1 -> Iq_Ref/1

== system power_dstatcom_pwm/DStatcom/Controller/Controller (sample time=Ts*32)/Current Regulator ==
  note: =================
  note: Current Regulators
  IdIq : Inport  PortDimensions=2
  IdIq_Ref : Inport  Port=2  PortDimensions=2
  Demux : Demux  Outputs=2
  Demux1 : Demux  Outputs=2
  Discrete Rate Limiter : powerlib_extras/Discrete  Control Blocks/Discrete Rate Limiter  R=240  F=-240  Vinit=0  Ts=Ts
  Id PID : powerlib_extras/Discrete  Control Blocks/Discrete PID Controller  Kp=Kp  Ki=Ki  Kd=Kd  TcD=TcD  Par_Limits=Par_Limits  Init=Init  Ts=Ts
  Id PID1 : powerlib_extras/Discrete  Control Blocks/Discrete PID Controller  Kp=Kp  Ki=Ki  Kd=Kd  TcD=TcD  Par_Limits=Par_Limits  Init=Init  Ts=Ts
  Mux : Mux  Inputs=2
  Sum : Sum  Inputs=|+-  SaturateOnIntegerOverflow=on  InputSameDT=on  OutDataTypeStr=Inherit: Same as first input
  Sum1 : Sum  Inputs=|+-  SaturateOnIntegerOverflow=on  InputSameDT=on  OutDataTypeStr=Inherit: Same as first input
  VdVq : Outport
  wires:
  Discrete Rate Limiter/1 -> Demux1/1
  IdIq_Ref/1 -> Discrete Rate Limiter/1
  Mux/1 -> VdVq/1
  Sum/1 -> Id PID/1
  Demux1/2 -> Sum1/2  "Iq_Ref"
  Sum1/1 -> Id PID1/1
  Demux/2 -> Sum1/1  "Iq"
  Demux1/1 -> Sum/2  "Id_Ref"
  Demux/1 -> Sum/1  "Id"
  Id PID/1 -> Mux/1  "Vd"
  Id PID1/1 -> Mux/2  "Vq"
  IdIq/1 -> Demux/1

== system power_dstatcom_pwm/DStatcom/Controller/Controller (sample time=Ts*32)/DC Voltage Regulator ==
  Vdc : Inport
  Vdc_Ref : Inport  Port=2
  -1<Id<+1 : Saturate  UpperLimit=1  LowerLimit=-1
  2250<Vdc<3750 : Saturate  UpperLimit=3750  LowerLimit=2250
  Discrete PI Controller : powerlib_extras/Discrete  Control Blocks/Discrete PI Controller  Kp=Kp  Ki=Ki  Par_Limits=[1 -1]  Init=0  Ts=Ts
  Discrete Rate Limiter1 : powerlib_extras/Discrete  Control Blocks/Discrete Rate Limiter  R=10000  F=-10000  Vinit=3000  Ts=Ts
  Sum : Sum  Inputs=|+-  SaturateOnIntegerOverflow=on  InputSameDT=on  OutDataTypeStr=Inherit: Same as first input
  Id_Ref : Outport  InitialOutput=0
  wires:
  Vdc_Ref/1 -> 2250<Vdc<3750/1
  2250<Vdc<3750/1 -> Discrete Rate Limiter1/1
  Sum/1 -> Discrete PI Controller/1
  Vdc/1 -> Sum/2
  Discrete Rate Limiter1/1 -> Sum/1
  Discrete PI Controller/1 -> -1<Id<+1/1
  -1<Id<+1/1 -> Id_Ref/1

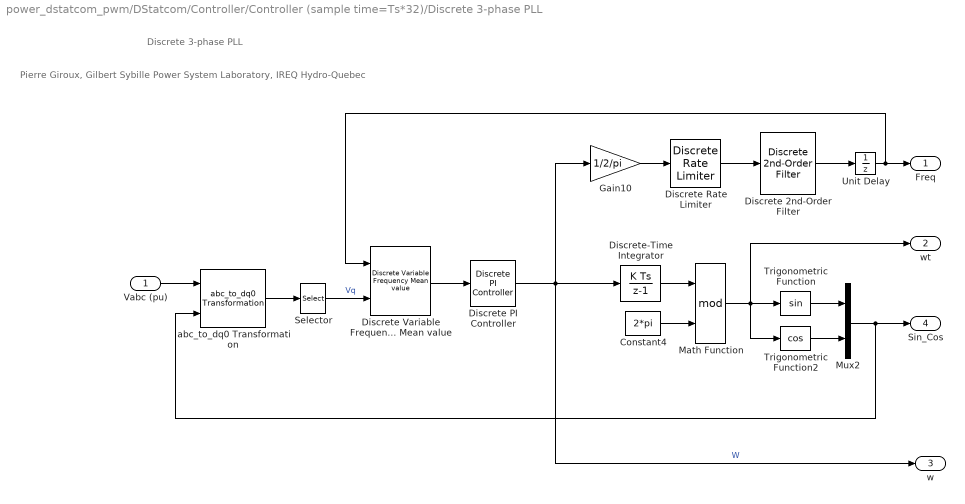
== system power_dstatcom_pwm/DStatcom/Controller/Controller (sample time=Ts*32)/Discrete 3-phase PLL ==
  note: Discrete 3-phase PLL
  note: Pierre Giroux, Gilbert Sybille
      | Power System Laboratory, IREQ
      | Hydro-Quebec
  Vabc (pu) : Inport  PortDimensions=3
  Constant4 : Constant  Value=2*pi
  Discrete PI Controller : powerlib_extras/Discrete  Control Blocks/Discrete PI Controller  Kp=Kp  Ki=Ki  Par_Limits=2*pi*Finit*[1.25 0.75]  Init=2*pi*Finit  Ts=Ts
  Discrete Rate Limiter : powerlib_extras/Discrete  Control Blocks/Discrete Rate Limiter  R=10  F=-10  Vinit=Finit  Ts=Ts
  Discrete Variable Frequency Mean value : powerlib_extras/Discrete Measurements/Discrete Variable Frequency Mean value  Finit=Finit  Fmin=45  Vinit=0  Ts=Ts
  Discrete 2nd-Order Filter : powerlib_extras/Discrete  Control Blocks/Discrete  2nd-Order Filter  FilterType=Lowpass  Fo=25  Zeta=0.707  Ts=Ts  Initialize=on  Vac_Init=[0 0 Finit]  Vdc_Init=Finit  PlotResponse=off  param1=[1 500 0.1]
  Discrete-Time Integrator : DiscreteIntegrator  InitialCondition=Phase_Init*pi/180  SampleTime=Ts  ICPrevOutput=DiscIntNeverNeededParam  ICPrevScaledInput=DiscIntNeverNeededParam
  Gain10 : Gain  Gain=1/2/pi  SaturateOnIntegerOverflow=on  OutDataTypeStr=Inherit: Same as input  ParamDataTypeStr=Inherit: Same as input
  Math Function : Math  Operator=mod  SaturateOnIntegerOverflow=on
  Mux2 : Mux  Inputs=2
  Selector : Selector  InputPortWidth=3  IndexOptions=Index vector (dialog)  Indices=2  OutputSizes=1
  Trigonometric Function : Trigonometry
  Trigonometric Function2 : Trigonometry  Operator=cos
  Unit Delay : UnitDelay  InitialCondition=Finit  SampleTime=Ts
  abc_to_dq0 Transformation : powerlib_extras/Measurements/abc_to_dq0 Transformation
  Freq : Outport
  wt : Outport  Port=2
  w : Outport  Port=3
  Sin_Cos : Outport  Port=4
  wires:
  Discrete Variable Frequency Mean value/1 -> Discrete PI Controller/1
  Vabc (pu)/1 -> abc_to_dq0 Transformation/1
  abc_to_dq0 Transformation/1 -> Selector/1
  Constant4/1 -> Math Function/2
  Discrete-Time Integrator/1 -> Math Function/1
  Math Function/1 -> Trigonometric Function/1, Trigonometric Function2/1, wt/1
  Trigonometric Function/1 -> Mux2/1
  Trigonometric Function2/1 -> Mux2/2
  Mux2/1 -> abc_to_dq0 Transformation/2, Sin_Cos/1
  Discrete PI Controller/1 -> w/1, Discrete-Time Integrator/1, Gain10/1  "W"
  Gain10/1 -> Discrete Rate Limiter/1
  Discrete Rate Limiter/1 -> Discrete 2nd-Order Filter/1
  Unit Delay/1 -> Freq/1, Discrete Variable Frequency Mean value/1
  Discrete 2nd-Order Filter/1 -> Unit Delay/1
  Selector/1 -> Discrete Variable Frequency Mean value/2  "Vq"

== system power_dstatcom_pwm/DStatcom/Controller/Controller (sample time=Ts*32)/Iq_ref (Manual) ==
  MagV : Inport  PortDimensions=1
  Qref : Inport  Port=2  PortDimensions=1
  -1<Iq<+1 : Saturate  UpperLimit=1  LowerLimit=-1
  Constant11 : Constant  Value=0
  Constant13 : Constant  Value=1e-6
  Deg->Rad1 : Gain  Gain=-1  SaturateOnIntegerOverflow=on  OutDataTypeStr=Inherit: Same as input  ParamDataTypeStr=Inherit: Same as input
  Discrete Rate Limiter : powerlib_extras/Discrete  Control Blocks/Discrete Rate Limiter  R=60*2  F=-60*2  Vinit=0  Ts=32*Ts
  Discrete 2nd-Order Filter : powerlib_extras/Discrete  Control Blocks/Discrete  2nd-Order Filter  FilterType=Lowpass  Fo=20  Zeta=0.707  Ts=32*Ts  Initialize=off  Vac_Init=[0.8 -25 60]  Vdc_Init=-0.4  PlotResponse=off  param1=[1 500 0.1]
  Product : Product  Inputs=*/  SaturateOnIntegerOverflow=on  InputSameDT=on  OutDataTypeStr=Inherit: Same as first input
  Relational Operator1 : RelationalOperator  Operator=~=  InputSameDT=on
  Switch : Switch  Threshold=0.5  SaturateOnIntegerOverflow=on  InputSameDT=on
  Iqref* : Outport
  wires:
  Discrete Rate Limiter/1 -> Product/1
  Qref/1 -> Discrete Rate Limiter/1
  -1<Iq<+1/1 -> Iqref*/1
  Deg->Rad1/1 -> -1<Iq<+1/1
  Product/1 -> Deg->Rad1/1
  Discrete 2nd-Order Filter/1 -> Product/2
  Switch/1 -> Discrete 2nd-Order Filter/1
  Constant13/1 -> Switch/3
  MagV/1 -> Switch/1, Relational Operator1/1
  Relational Operator1/1 -> Switch/2
  Constant11/1 -> Relational Operator1/2

== system power_dstatcom_pwm/DStatcom/Controller/Controller (sample time=Ts*32)/Measuremnt Unit ==
  sin_cos : Inport
  Vabc : Inport  Port=2
  Iabc : Inport  Port=3
  Imeas : powerlib_extras/Measurements/abc_to_dq0 Transformation
  "Mag_V " : Fcn  Expr=sqrt(u[1]*u[1]+u[2]*u[2])
  Selector : Selector  InputPortWidth=3  IndexOptions=Index vector (dialog)  Indices=[1 2]  OutputSizes=1
  Selector1 : Selector  InputPortWidth=3  IndexOptions=Index vector (dialog)  Indices=[1 2]  OutputSizes=1
  Vmeas : powerlib_extras/Measurements/abc_to_dq0 Transformation
  IdIq : Outport
  MagV : Outport  Port=2
  tag scope: IdIq=global, VdVq=global
  wires:
  "Mag_V "/1 -> MagV/1
  Selector1/1 -> [IdIq], IdIq/1
  Selector/1 -> "Mag_V "/1, [VdVq]
  Imeas/1 -> Selector1/1
  Iabc/1 -> Imeas/1
  sin_cos/1 -> Imeas/2, Vmeas/2
  Vmeas/1 -> Selector/1
  Vabc/1 -> Vmeas/1

== system power_dstatcom_pwm/DStatcom/Controller/Controller (sample time=Ts*32)/Vd_Vq--> m,Phi ==
  VdVq : Inport
  Fcn3 : Fcn  Expr=sqrt(u[1]*u[1]+u[2]*u[2])
  Fcn4 : Fcn  Expr=atan2(u[2]+1e-6,u[1])*180/pi
  Mux2 : Mux  Inputs=2
  m_Phi : Outport
  wires:
  Fcn4/1 -> Mux2/2
  Mux2/1 -> m_Phi/1
  Fcn3/1 -> Mux2/1
  VdVq/1 -> Fcn4/1, Fcn3/1

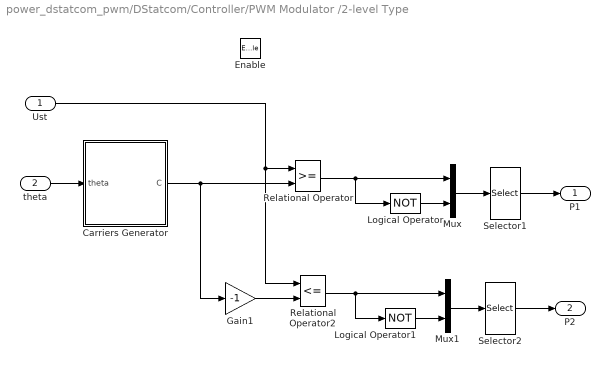
== system power_dstatcom_pwm/DStatcom/Controller/PWM Modulator /2-level Type ==
  Ust : Inport
  theta : Inport  Port=2
  Enable : EnablePort  PropagateVarSize=During execution
  Carriers Generator : Subsystem
  Gain1 : Gain  Gain=-1  SaturateOnIntegerOverflow=on  OutDataTypeStr=Inherit: Same as input  ParamDataTypeStr=Inherit: Same as input
  Logical Operator : Logic  Operator=NOT
  Logical Operator1 : Logic  Operator=NOT
  Mux : Mux  Inputs=[3 3]
  Mux1 : Mux  Inputs=[3 3]
  Relational Operator : RelationalOperator  InputSameDT=on
  Relational Operator2 : RelationalOperator  Operator=<=  InputSameDT=on
  Selector1 : Selector  InputPortWidth=6  IndexOptions=Index vector (dialog)  Indices=[1 4 2 5 3 6]  OutputSizes=1
  Selector2 : Selector  InputPortWidth=6  IndexOptions=Index vector (dialog)  Indices=[1 4 2 5 3 6]  OutputSizes=1
  P1 : Outport
  P2 : Outport  Port=2
  wires:
  Selector2/1 -> P2/1
  Mux1/1 -> Selector2/1
  Logical Operator1/1 -> Mux1/2
  Relational Operator2/1 -> Logical Operator1/1, Mux1/1
  Selector1/1 -> P1/1
  Mux/1 -> Selector1/1
  Logical Operator/1 -> Mux/2
  Gain1/1 -> Relational Operator2/2
  Carriers Generator/1(C) -> Relational Operator/2, Gain1/1
  Relational Operator/1 -> Mux/1, Logical Operator/1
  theta/1 -> Carriers Generator/1(theta)
  Ust/1 -> Relational Operator2/1, Relational Operator/1

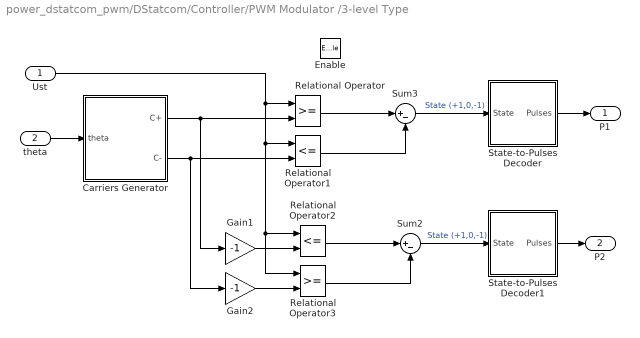
== system power_dstatcom_pwm/DStatcom/Controller/PWM Modulator /3-level Type ==
  Ust : Inport
  theta : Inport  Port=2
  Enable : EnablePort  PropagateVarSize=During execution
  Carriers Generator : Subsystem
  Gain1 : Gain  Gain=-1  SaturateOnIntegerOverflow=on  OutDataTypeStr=Inherit: Same as input  ParamDataTypeStr=Inherit: Same as input
  Gain2 : Gain  Gain=-1  SaturateOnIntegerOverflow=on  OutDataTypeStr=Inherit: Same as input  ParamDataTypeStr=Inherit: Same as input
  Relational Operator : RelationalOperator  InputSameDT=on
  Relational Operator1 : RelationalOperator  Operator=<=  InputSameDT=on
  Relational Operator2 : RelationalOperator  Operator=<=  InputSameDT=on
  Relational Operator3 : RelationalOperator  InputSameDT=on
  State-to-Pulses Decoder : Subsystem
  State-to-Pulses Decoder1 : Subsystem
  Sum2 : Sum  Inputs=|+-  SaturateOnIntegerOverflow=on  InputSameDT=on  OutDataTypeStr=Inherit: Same as first input
  Sum3 : Sum  Inputs=|+-  SaturateOnIntegerOverflow=on  InputSameDT=on  OutDataTypeStr=Inherit: Same as first input
  P1 : Outport
  P2 : Outport  Port=2
  wires:
  Ust/1 -> Relational Operator1/1, Relational Operator2/1, Relational Operator3/1, Relational Operator/1
  State-to-Pulses Decoder1/1(Pulses) -> P2/1
  theta/1 -> Carriers Generator/1(theta)
  State-to-Pulses Decoder/1(Pulses) -> P1/1
  Relational Operator/1 -> Sum3/1
  Relational Operator1/1 -> Sum3/2
  Carriers Generator/1(C+) -> Relational Operator/2, Gain1/1
  Carriers Generator/2(C-) -> Relational Operator1/2, Gain2/1
  Relational Operator2/1 -> Sum2/1
  Relational Operator3/1 -> Sum2/2
  Gain1/1 -> Relational Operator2/2
  Gain2/1 -> Relational Operator3/2
  Sum3/1 -> State-to-Pulses Decoder/1(State)  "State (+1,0,-1)"
  Sum2/1 -> State-to-Pulses Decoder1/1(State)  "State (+1,0,-1)"

== system power_dstatcom_pwm/DStatcom/Controller/PWM Modulator /Internal ==
  Constant1 : Constant  Value=[0 -2*pi/3 2*pi/3]
  Constant6 : Constant  Value=Phase
  Constant7 : Constant  Value=2*pi
  Constant8 : Constant  Value=Freq
  Constant9 : Constant  Value=m
  Product1 : Product  Inputs=3  SaturateOnIntegerOverflow=on  InputSameDT=on  OutDataTypeStr=Inherit: Same as first input
  Product2 : Product  SaturateOnIntegerOverflow=on  InputSameDT=on  OutDataTypeStr=Inherit: Same as first input
  Sum4 : Sum  Inputs=+++  SaturateOnIntegerOverflow=on  InputSameDT=on  OutDataTypeStr=Inherit: Same as first input
  Trigonometric Function1 : Trigonometry
  deg. ->rad : Gain  Gain=pi/180  SaturateOnIntegerOverflow=on  OutDataTypeStr=Inherit: Same as input  ParamDataTypeStr=Inherit: Same as input
  "t " : DigitalClock  SampleTime=Ts
  Ust : Outport
  wires:
  Constant7/1 -> Product1/1
  Constant8/1 -> Product1/2
  "t "/1 -> Product1/3
  Product1/1 -> Sum4/1
  Constant1/1 -> Sum4/2
  Constant6/1 -> deg. ->rad/1
  deg. ->rad/1 -> Sum4/3
  Sum4/1 -> Trigonometric Function1/1
  Trigonometric Function1/1 -> Product2/2
  Constant9/1 -> Product2/1
  Product2/1 -> Ust/1

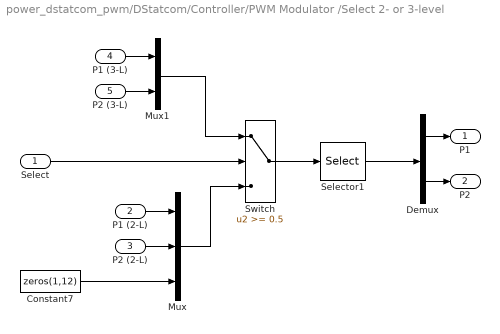
== system power_dstatcom_pwm/DStatcom/Controller/PWM Modulator /Select 2- or 3-level ==
  Select : Inport  PortDimensions=1
  P1 (2-L) : Inport  Port=2  PortDimensions=6
  P2 (2-L) : Inport  Port=3  PortDimensions=6
  P1 (3-L) : Inport  Port=4  PortDimensions=12
  P2 (3-L) : Inport  Port=5  PortDimensions=12
  Constant7 : Constant  Value=zeros(1,12)
  Demux : Demux  Outputs=[nPulses nPulses]
  Mux : Mux  Inputs=[6 6 12]
  Mux1 : Mux  Inputs=[12 12]
  Selector1 : Selector  InputPortWidth=24  IndexOptions=Index vector (dialog)  Indices=SelectorElements  OutputSizes=1
  Switch : Switch  Threshold=0.5  SaturateOnIntegerOverflow=on  InputSameDT=on
  P1 : Outport
  P2 : Outport  Port=2
  wires:
  Mux/1 -> Switch/3
  P2 (3-L)/1 -> Mux1/2
  P1 (3-L)/1 -> Mux1/1
  Demux/2 -> P2/1
  Select/1 -> Switch/2
  Demux/1 -> P1/1
  P2 (2-L)/1 -> Mux/2
  P1 (2-L)/1 -> Mux/1
  Constant7/1 -> Mux/3
  Mux1/1 -> Switch/1
  Selector1/1 -> Demux/1
  Switch/1 -> Selector1/1
